simulink model "AL_AL_FMU"  (R2023b)
settings: Solver=FixedStepDiscrete  StartTime=0.0  StopTime=1730  FixedStep=1  RelTol=1e-3
settings Model: Creator=angel  LastModifiedBy=Symvoulos_OSE

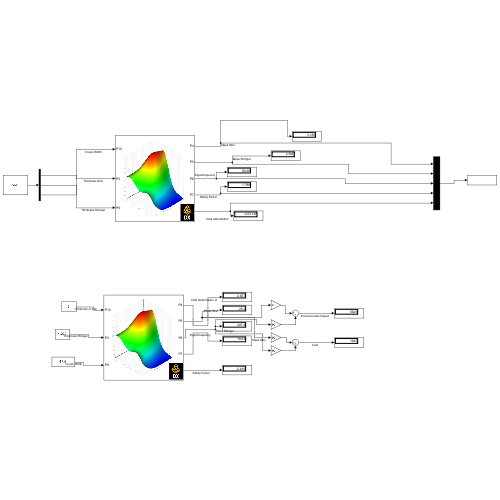
[thumbnail: Simulink's stored preview of the top-level diagram]
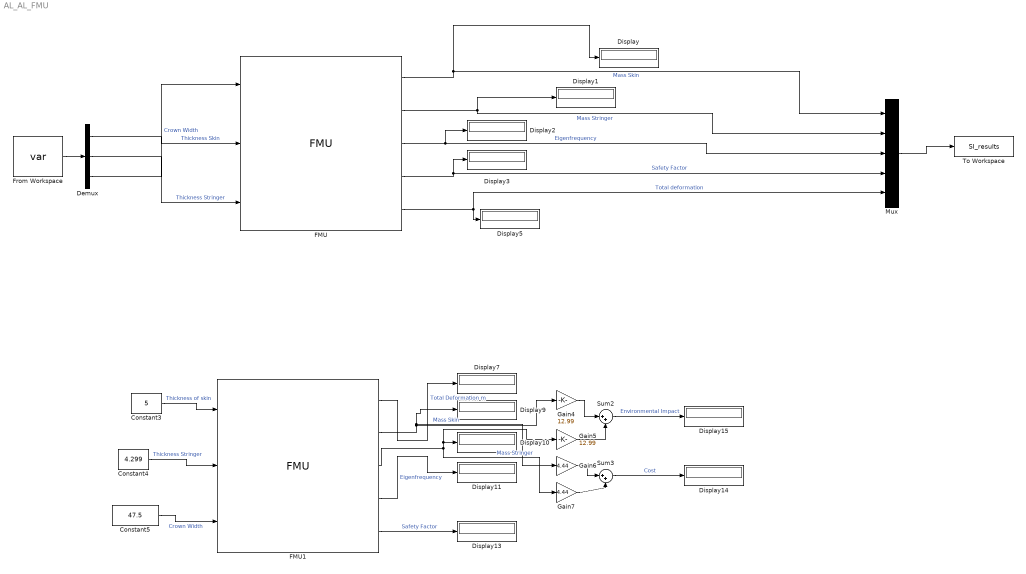
== system AL_AL_FMU ==
  Constant3 : Constant  Value=5
  Constant4 : Constant  Value=4.299
  Constant5 : Constant  Value=47.5
  Demux : Demux  Outputs=3
  Display{,1..3,5,7,9..11,13..15} (12 alike) : Display
  FMU : FMU  FMUName=AL_AL.fmu  FMUMode=ModelExchange  FMUInitializeEnumObject=off  FMUCachedDialogLayout="{\"Geometry\":[2953,164,505,426],\"ParameterColumnsWidthConfig\":\"{\\\"columns\\\":[{\\\"name\\\":\\\"Parameter\\\",\\\"width\\\":171},{\\\"name\\\":\\\"Value\\\",\\\"width\\\":135},{\\\"name\\\":\\\"Unit\\\",\\\"width\\\":125},{\\\"name\\\":\\\"Description\\\",\\\"width\\\":180}]}\",\"InputColumnsWidthConfig\":[],\"OutputColumnsWidthConfig\":[]}"
      settings: MultithreadedSim=off
      mask Type: Ansys DesignXplorer Response Surface [Model Exchange, v2.0]
      mask Display:
      | if (exist([Simulink.fileGenControl('get','CacheFolder') '\slprj\_fmu\4d5ba8aa6d2f98916561d2ac241f056d\AL_AL\model.png'],'file'))
      |     image([Simulink.fileGenControl('get','CacheFolder') '\slprj\_fmu\4d5ba8aa6d2f98916561d2ac241f056d\AL_AL\model.png']);
      | else
      |     disp('Ansys DesignXplorer Response Surface');
      | end
      | port_label('output',1,'P4');
      | port_label('output',2,'P5');
      | port_label('output',3,'P6');
      | port_label('output',4,'P7');
      | port_label('output',5,'P8');
      | port_label('input',1,'P10');
      | port_label('input',2,'P3');
      | port_label('input',3,'P9');
  FMU1 : FMU  FMUName=al_al.fmu  FMUMode=ModelExchange  FMUInitializeEnumObject=off  FMUCachedDialogLayout="{\"Geometry\":[754,402,505,426],\"ParameterColumnsWidthConfig\":\"{\\\"columns\\\":[{\\\"name\\\":\\\"Parameter\\\",\\\"width\\\":171},{\\\"name\\\":\\\"Value\\\",\\\"width\\\":135},{\\\"name\\\":\\\"Unit\\\",\\\"width\\\":125},{\\\"name\\\":\\\"Description\\\",\\\"width\\\":180}]}\",\"InputColumnsWidthConfig\":\"{\\\"columns\\\":[{\\\"name\\\":\\\"Name\\\",\\\"width\\\":127},{\\\"name\\\":\\\"Visibility\\\",\\\"width\\\":79},{\\\"name\\\":\\\"Start\\\",\\\"width\\\":116},{\\\"name\\\":\\\"Unit\\\",\\\"width\\\":113},{\\\"name\\\":\\\"Type Object\\\",\\\"width\\\":172}]}\",\"OutputColumnsWidthConfig\":\"{\\\"columns\\\":[{\\\"name\\\":\\\"Name\\\",\\\"width\\\":127},{\\\"name\\\":\\\"Visibility\\\",\\\"width\\\":79},{\\\"name\\\":\\\"Start\\\",\\\"width\\\":116},{\\\"name\\\":\\\"Unit\\\",\\\"width\\\":113},{\\\"name\\\":\\\"Type Object\\\",\\\"width\\\":172}]}\"}"
      settings: MultithreadedSim=off
      mask Type: Ansys DesignXplorer Response Surface [Model Exchange, v2.0]
      mask Display:
      | if (exist([Simulink.fileGenControl('get','CacheFolder') '\slprj\_fmu\eac813e31f0c5e3bb6a5e3a40d4e5b0e\al_al\model.png'],'file'))
      |     image([Simulink.fileGenControl('get','CacheFolder') '\slprj\_fmu\eac813e31f0c5e3bb6a5e3a40d4e5b0e\al_al\model.png']);
      | else
      |     disp('Ansys DesignXplorer Response Surface');
      | end
      | port_label('output',1,'P4');
      | port_label('output',2,'P5');
      | port_label('output',3,'P6');
      | port_label('output',4,'P7');
      | port_label('output',5,'P8');
      | port_label('input',1,'P10');
      | port_label('input',2,'P3');
      | port_label('input',3,'P9');
  From Workspace : FromWorkspace  VariableName=var  SampleTime=1
  Gain4 : Gain  Gain=12.99
  Gain5 : Gain  Gain=12.99
  Gain6 : Gain  Gain=4.44
  Gain7 : Gain  Gain=4.44
  Mux : Mux  Inputs=5
  Sum2 : Sum  Inputs=|++
  Sum3 : Sum  Inputs=|++
  To Workspace : ToWorkspace  VariableName=SI_results  SaveFormat=Structure  SampleTime=-1
  wires:
  FMU/1 -> Display/1, Mux/1  "Mass Skin"
  FMU/2 -> Mux/2, Display1/1  "Mass Stringer"
  FMU/3 -> Display2/1, Mux/3  "Eigenfrequency"
  FMU/4 -> Display3/1, Mux/4  "Safety Factor"
  FMU/5 -> Display5/1, Mux/5  "Total deformation"
  Demux/3 -> FMU/1  "Crown Width"
  Demux/1 -> FMU/2  "Thickness Skin"
  Demux/2 -> FMU/3  "Thickness Stringer"
  Sum3/1 -> Display14/1  "Cost"
  Gain7/1 -> Sum3/2
  Gain6/1 -> Sum3/1
  Sum2/1 -> Display15/1  "Environmental Impact"
  Gain5/1 -> Sum2/2
  Gain4/1 -> Sum2/1
  Constant5/1 -> FMU1/3  "Crown Width"
  Constant4/1 -> FMU1/2  "Thickness Stringer"
  Constant3/1 -> FMU1/1  "Thickness of skin"
  FMU1/5 -> Display13/1  "Safety Factor"
  FMU1/4 -> Display11/1  "Eigenfrequency"
  FMU1/3 -> Gain7/1, Display10/1, Gain5/1  "Mass Stringer"
  FMU1/2 -> Display9/1, Gain6/1, Gain4/1  "Mass Skin"
  FMU1/1 -> Display7/1  "Total Deformation m"
  From Workspace/1 -> Demux/1
  Mux/1 -> To Workspace/1
